simulink model "Project_PV"  (R2024a)
settings: Solver=VariableStepAuto  StartTime=0.0  StopTime=3  RelTol=1e-3
undefined symbols (not defined in the file): Ion, Lithium
libraries: spsSeriesRLCBranchLib x4, spsCurrentMeasurementLib x2, spsIdealSwitchLib x2, spsVoltageMeasurementLib x2, spsBatteryLib x1, simulink x1, spsDiodeLib x1, spsMosfetLib x1, spsOnDelayLib x1, spsPVArrayLib x1, sps_lib x1
settings Model: Creator=vivek  LastModifiedBy=vivek

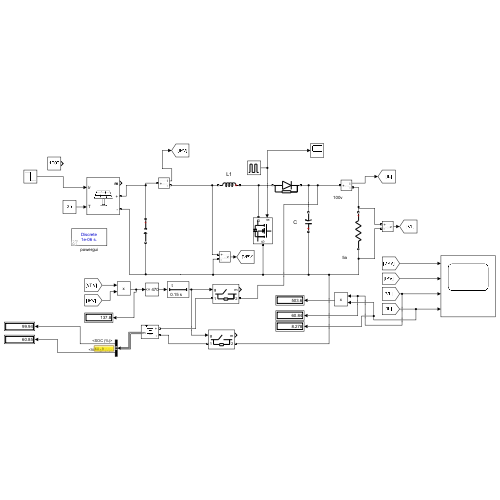
[thumbnail: Simulink's stored preview of the top-level diagram]
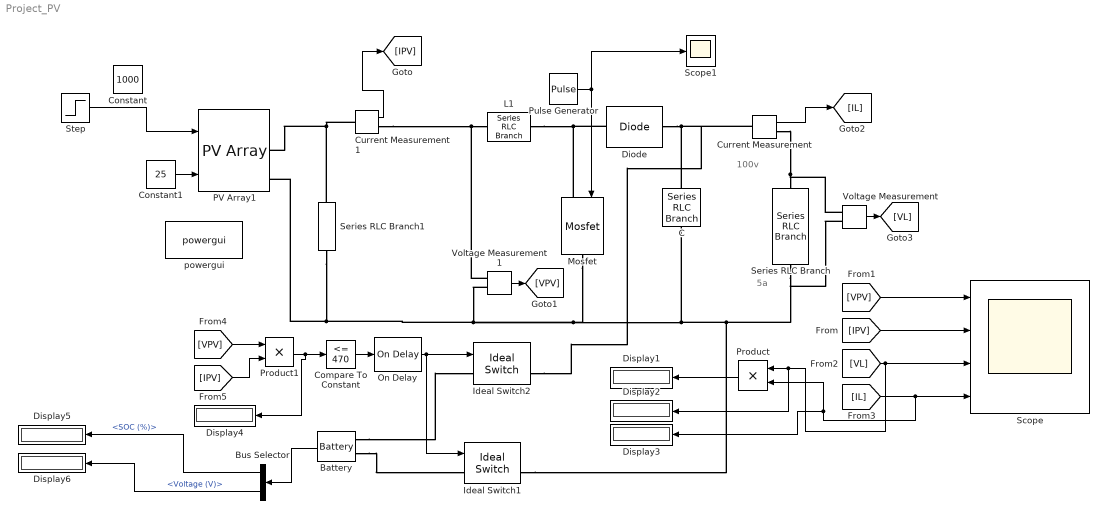
== system Project_PV ==
  note: 5a
  note: 100v
  Battery : spsBatteryLib/Battery  BatType=Lithium-Ion  ShowTempParam=off  ThermalPreset=no  ShowAgeParam=off  NomV=53.1  NomQ=5.4  SOC=100  Batt_Tr=0.15  PresetModel=on  MaxQ=5.4  MinV=39  FullV=60.5273  Dis_rate=2.3478  R=0.096296  Normal_OP=4.8835  expZone="[56.1801     0.265304]"  current=[6.5 13 32.5]  Units=Time  Tci=20  NomT=20  T2=-30  MaxQ2=4.8  FullV2=7.1  Normal_OP2=5.655  expZone2="[6.58           1]"  Rca=0.6  ti=2000  Dp=0  Neq0=0  Tsim=1e6  Ta1=25  Qeol=5.4*0.9  Reol=0.013333*1.2  Char_age=[2.3478, 3]  Dis_age=[2.3478, 10]  N1=1500  N2=10500  N3=1000  N4=1400  Ta2=45  N5=950
  Bus Selector : BusSelector  OutputSignals=SOC (%),Voltage (V)
  C : spsSeriesRLCBranchLib/Series RLC Branch  LConnTagsString=__new0  RConnTagsString=__new0  BranchType=C  Resistance=1e-4  Inductance=200e-6  SetiL0=off  InitialCurrent=0  Capacitance=2000e-6  Setx0=off  InitialVoltage=7.5  Measurements=None
  Compare To Constant : simulink/Logic and Bit Operations/Compare To Constant  relop=<=  const=470  OutDataTypeStr=boolean  ZeroCross=off
  Constant : Constant  Value=1000
  Constant1 : Constant  Value=25
  Current Measurement : spsCurrentMeasurementLib/Current Measurement  PhasorSimulation=off  OutputType=Complex  PSBequivalent=0
  Current Measurement1 : spsCurrentMeasurementLib/Current Measurement  PhasorSimulation=off  OutputType=Complex  PSBequivalent=0
  Diode : spsDiodeLib/Diode  Ron=0.001  Lon=0  Vf=0.8  IC=0  UseSnubber=0  Rs=500  Cs=250e-9  Measurements=off
  Display{1..6} (6 alike) : Display
  Ideal Switch1 : spsIdealSwitchLib/Ideal Switch  Ron=0.001  Lon=0  IC=0  Rs=1e5  Cs=inf  Measurements=on
  Ideal Switch2 : spsIdealSwitchLib/Ideal Switch  Ron=0.001  Lon=0  IC=0  Rs=1e5  Cs=inf  Measurements=on
  L1 : spsSeriesRLCBranchLib/Series RLC Branch  LConnTagsString=__new0  RConnTagsString=__new0  BranchType=L  Resistance=1e-4  Inductance=6.09e-3  SetiL0=off  InitialCurrent=14  Capacitance=30e-6  Setx0=off  InitialVoltage=150  Measurements=None
  Mosfet : spsMosfetLib/Mosfet  Ron=0.1  Lon=0  Rd=0.01  Vfd=0  IC=0  Rs=1e5  Cs=inf  Measurements=off
  On Delay : spsOnDelayLib/On Delay  DelayType=On delay  delay=0.15  ic=0  Ts=0
  PV Array1 : spsPVArrayLib/PV Array  Npar=5  Nser=1  PlotType=array @ 1000 W/m2 & specified temperatures  S_vec="[ 1000  500  100 ]"  Temp_C_vec="[ 45 25  ]"  ModuleName=User-defined  PlotWhenSelected=off  Pm=213.15  Ncell=60  Voc=36.3  Isc=7.84  Vm=29  Im=7.35  beta_Voc_pc=-0.36099  alpha_Isc_pc=0.102  beta_Voc=-0.13104  alpha_Isc=0.0079968  IL=7.8654  I0=2.9273e-10  nI=0.98119  Rsh=313.0553  Rs=0.39381  RobustModel=off  RobustCellTemperature=313.3991  BAL=on  Tc=1e-6  Tfilter=5e-5
  Product : Product
  Product1 : Product
  Pulse Generator : DiscretePulseGenerator  PulseType=Time based  Period=1/20000  PulseWidth=46
  Scope : Scope  NumInputPorts=4
  Scope1 : Scope
  Series RLC Branch : spsSeriesRLCBranchLib/Series RLC Branch  LConnTagsString=__new0  RConnTagsString=__new0  BranchType=R  Resistance=7.35  Inductance=1e-3  SetiL0=off  InitialCurrent=0  Capacitance=1e-6  Setx0=off  InitialVoltage=0  Measurements=None
  Series RLC Branch1 : spsSeriesRLCBranchLib/Series RLC Branch  LConnTagsString=__new0  RConnTagsString=__new0  BranchType=C  Resistance=1  Inductance=1e-3  SetiL0=off  InitialCurrent=0  Capacitance=70e-5  Setx0=off  InitialVoltage=0  Measurements=None
  Step : Step  Before=1000  After=300  SampleTime=0
  Voltage Measurement : spsVoltageMeasurementLib/Voltage Measurement  PhasorSimulation=off  OutputType=Complex  PSBequivalent=0
  Voltage Measurement1 : spsVoltageMeasurementLib/Voltage Measurement  PhasorSimulation=off  OutputType=Complex  PSBequivalent=0
  powergui : sps_lib/powergui  Priority=1  SimulationMode=Discrete  SampleTime=1e-6  frequency=60  Iterations=50  frequencyindice=0  Pbase=100e6  ErrMax=1e-4  UnitsV=kV  UnitsW=MW  buscounter=0  FunctionMessages=off  echomessages=off  EnableUseOfTLC=off  CurrentSourceSwitches=off  DisableSnubberDevices=off  DisableRonSwitches=off  DisableVfSwitches=off  DisplayEquations=off  AutomaticDiscreteSolvers=off  SolverType=Tustin/Backward Euler (TBE)  Interpol=off  ExternalGateDelay=off  methode=off  Ts=100  x0status=blocks  SPID=on  SwTol=0  HookPort=off  NonlinearTolerance=1e-4  nMaxIteration=100  ContinueOnMaxIteration=off  RestoreLinks=warning  ResistiveCurrentMeasurement=off  Frange=[0:2:500]  Ylog=off  Xlog=on  ShowGrid=off  save=off  variable=ZData  structure=0  ZoomFFT=off  StartTime=0.0  cycles=1  DisplayStyle=1  fundamental=60  FreqAxis=off  MaxFrequency=1000  frequencyindicesteady=1  RmsSteady=1  display=off
  wires:
  Constant1/1 -> PV Array1/2
  Voltage Measurement1/1 -> [VPV]
  [IPV] -> Scope/2
  [VPV] -> Scope/1
  Pulse Generator/1 -> Scope1/1, Mosfet/1
  Current Measurement/1 -> [IL]
  Voltage Measurement/1 -> [VL]
  [VL] -> Display2/1, Product/1, Scope/3
  [IL] -> Display3/1, Product/2, Scope/4
  Product/1 -> Display1/1
  Current Measurement1/1 -> [IPV]
  [VPV] -> Product1/1
  [IPV] -> Product1/2
  Product1/1 -> Display4/1, Compare To Constant/1
  Battery/1 -> Bus Selector/1
  Bus Selector/2 -> Display6/1  "<Voltage (V)>"
  Bus Selector/1 -> Display5/1  "<SOC (%)>"
  Compare To Constant/1 -> On Delay/1
  Step/1 -> PV Array1/1
  On Delay/1 -> Ideal Switch2/1, Ideal Switch1/1
  connections:
  Voltage Measurement1/LConn1 -- Current Measurement1/RConn1 -- L1/RConn1
  Voltage Measurement/LConn1 -- Current Measurement/RConn1 -- Series RLC Branch/LConn1
  L1/LConn1 -- Diode/LConn1 -- Mosfet/LConn1
  C/RConn1 -- Ideal Switch2/RConn1 -- Current Measurement/LConn1 -- Diode/RConn1
  Mosfet/RConn1 -- Ideal Switch1/RConn1 -- Voltage Measurement/LConn2 -- Series RLC Branch/RConn1 -- C/LConn1 -- Voltage Measurement1/LConn2 -- Series RLC Branch1/RConn1 -- PV Array1/RConn2
  Series RLC Branch1/LConn1 -- Current Measurement1/LConn1 -- PV Array1/RConn1
  Battery/LConn2 -- Ideal Switch1/LConn1
  Battery/LConn1 -- Ideal Switch2/LConn1
